simulink model "Linearsystem"  (R2018b)
settings: Solver=ode4  StartTime=0.0  StopTime=10  FixedStep=0.02  RelTol=1e-3
InitFcn:
  | loadmatfile;
StopFcn:
  | linear_verification_plot;
undefined symbols (not defined in the file or in its folder): A, B, C, D
settings Model: Creator=arthus  LastModifiedBy=arthus

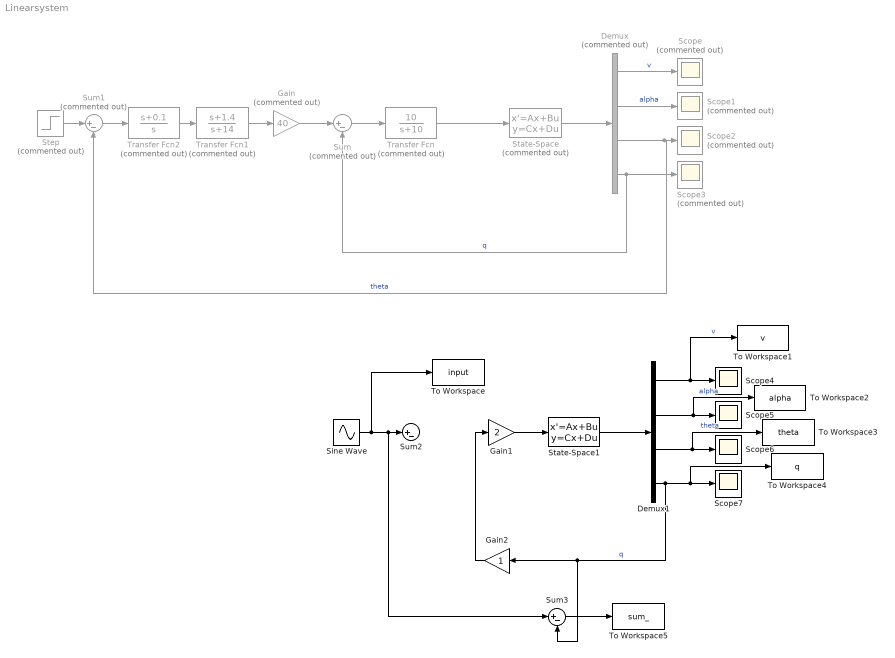
== system Linearsystem ==
  Demux : Demux  Commented=on
  Demux1 : Demux
  Gain : Gain  Commented=on  Gain=40
  Gain1 : Gain  Gain=2
  Gain2 : Gain
  Scope{,1..3} (4 alike) : Scope  Commented=on
  Scope{4..7} (4 alike) : Scope
  Sine Wave : Sin  Frequency=pi  SampleTime=0
  State-Space : StateSpace  Commented=on  A=A  B=B  C=C  D=D  InitialCondition=0
  State-Space1 : StateSpace  A=A  B=B  C=C  D=D  InitialCondition=[0 1 0 0]
  Step : Step  Commented=on  Time=0  SampleTime=0
  Sum : Sum  Commented=on  Inputs=|+-
  Sum1 : Sum  Commented=on  Inputs=|+-
  Sum2 : Sum  Inputs=|+-
  Sum3 : Sum  Inputs=|+-
  To Workspace : ToWorkspace  VariableName=input  SaveFormat=Timeseries  SampleTime=-1
  To Workspace1 : ToWorkspace  VariableName=v  SampleTime=-1
  To Workspace2 : ToWorkspace  VariableName=alpha  SampleTime=-1
  To Workspace3 : ToWorkspace  VariableName=theta  SampleTime=-1
  To Workspace4 : ToWorkspace  VariableName=q  SampleTime=-1
  To Workspace5 : ToWorkspace  VariableName=sum_  SampleTime=-1
  Transfer Fcn : TransferFcn  Commented=on  Numerator=[10]  Denominator=[1 10]
  Transfer Fcn1 : TransferFcn  Commented=on  Numerator=[1 1.4]  Denominator=[1 14]
  Transfer Fcn2 : TransferFcn  Commented=on  Numerator=[1 0.1]  Denominator=[1 0]
  wires:
  Sum/1 -> Transfer Fcn/1
  State-Space/1 -> Demux/1
  Demux/1 -> Scope/1  "v"
  Demux/2 -> Scope1/1  "alpha"
  Demux/3 -> Sum1/2, Scope2/1  "theta"
  Demux/4 -> Scope3/1, Sum/2  "q"
  Gain/1 -> Sum/1
  Transfer Fcn1/1 -> Gain/1
  Transfer Fcn2/1 -> Transfer Fcn1/1
  Step/1 -> Sum1/1
  Sum1/1 -> Transfer Fcn2/1
  Transfer Fcn/1 -> State-Space/1
  Demux1/1 -> To Workspace1/1, Scope4/1  "v"
  Demux1/3 -> To Workspace3/1, Scope6/1  "theta"
  Demux1/4 -> Sum3/2, Gain2/1, To Workspace4/1, Scope7/1  "q"
  Demux1/2 -> To Workspace2/1, Scope5/1  "alpha"
  State-Space1/1 -> Demux1/1
  Gain1/1 -> State-Space1/1
  Sine Wave/1 -> To Workspace/1, Sum3/1, Sum2/1
  Sum3/1 -> To Workspace5/1
  Gain2/1 -> Gain1/1
